simulink model "modulator_resonant_LLC"  (R2025b)
settings: Solver=VariableStepAuto  StartTime=0.0  StopTime=10.0  RelTol=1e-3
values from neighbouring files (symbols this model uses):
  fres = fPWM_DAB    (= 25000)    [init_model.m]
  tc = ts_dab/10    (= 4e-06)    [init_model.m]
settings Model: Creator=dbagn  LastModifiedBy=dbagn

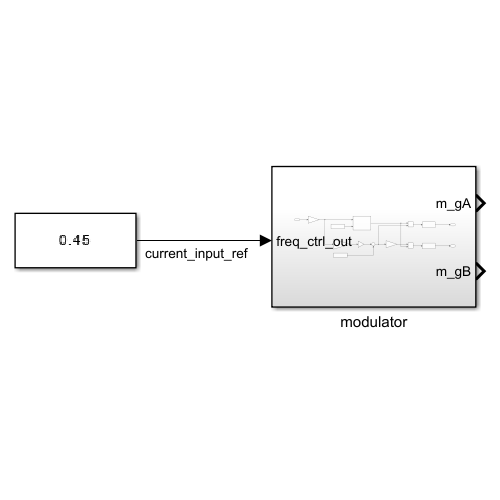
[thumbnail: Simulink's stored preview of the top-level diagram]
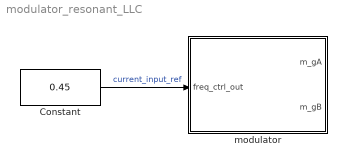
== system modulator_resonant_LLC ==
  Constant : Constant  Value=0.45
  modulator : Subsystem
  wires:
  Constant/1 -> modulator/1(freq_ctrl_out)  "current_input_ref"

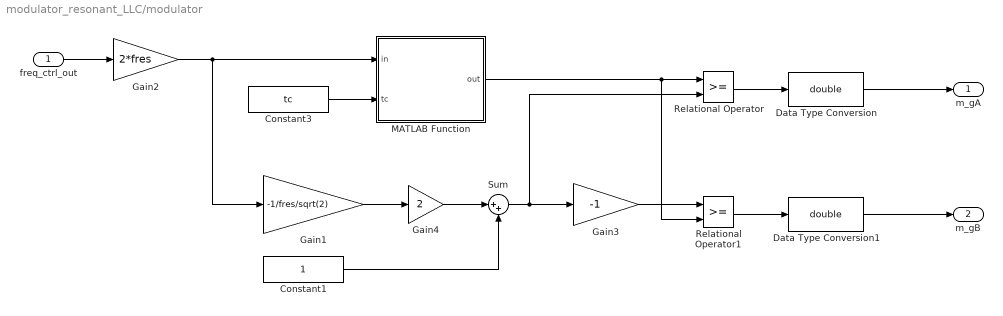
== system modulator_resonant_LLC/modulator ==
  freq_ctrl_out : Inport
  Constant1 : Constant
  Constant3 : Constant  Value=tc
  Data Type Conversion : DataTypeConversion  OutDataTypeStr=double  SaturateOnIntegerOverflow=off  RndMeth=Floor
  Data Type Conversion1 : DataTypeConversion  OutDataTypeStr=double  SaturateOnIntegerOverflow=off  RndMeth=Floor
  Gain1 : Gain  Gain=-1/fres/sqrt(2)  OutDataTypeStr=double
  Gain2 : Gain  Gain=2*fres  OutDataTypeStr=double
  Gain3 : Gain  Gain=-1  OutDataTypeStr=double
  Gain4 : Gain  Gain=2  OutDataTypeStr=double
  MATLAB Function : MATLAB Function  TreatAsAtomicUnit=on  SystemSampleTime=tc
  Relational Operator : RelationalOperator
  Relational Operator1 : RelationalOperator
  Sum : Sum  Inputs=|++
  m_gA : Outport
  m_gB : Outport  Port=2
  wires:
  freq_ctrl_out/1 -> Gain2/1
  MATLAB Function/1(out) -> Relational Operator1/2, Relational Operator/1
  Constant3/1 -> MATLAB Function/2(tc)
  Relational Operator/1 -> Data Type Conversion/1
  Data Type Conversion/1 -> m_gA/1
  Data Type Conversion1/1 -> m_gB/1
  Gain2/1 -> Gain1/1, MATLAB Function/1(in)
  Gain1/1 -> Gain4/1
  Sum/1 -> Gain3/1, Relational Operator/2
  Constant1/1 -> Sum/2
  Gain3/1 -> Relational Operator1/1
  Relational Operator1/1 -> Data Type Conversion1/1
  Gain4/1 -> Sum/1

== matlab function modulator_resonant_LLC/modulator/MATLAB Function ==
  data: in input; out output; tc input
function out = triangle(in,tc)

persistent y k

if isempty(y)
    y = 0;
    k = 1;
end

if y > 1
    k = -1;
    y = y + 4*k * in * tc;
elseif y < -1
    k = 1;
    y = y + 4*k * in * tc;
else
    y = y + 4*k * in * tc;
end
out = y;
